simulink model "SolarPackBuckConverter"  (R2024b)
settings: Solver=VariableStepAuto  StartTime=0.0  StopTime=0.1  RelTol=1e-3
values from neighbouring files (symbols this model uses):
  C1_actual = 470e-6    (= 0.00047)    [Buck_Design.m]
  C1_esr = 50e-3    (= 0.05)    [Buck_Design.m]
  C2_actual = 470e-6    (= 0.00047)    [Buck_Design.m]
  C2_esr = 50e-3    (= 0.05)    [Buck_Design.m]
  D1 = Vstage / Vg    (= 0.190476190476)    [Buck_Design.m]
  D2 = V / Vstage    (= 0.175)    [Buck_Design.m]
  L1_actual = 270e-6    (= 0.00027)    [Buck_Design.m]
  L1_esr = 14e-3    (= 0.014)    [Buck_Design.m]
  L2_actual = 12e-6    (= 1.2e-05)    [Buck_Design.m]
  L2_esr = 2.08e-3    (= 0.00208)    [Buck_Design.m]
  Rbat = 0.008    [Buck_Design.m]
  Rlimit = 0.1    [Buck_Design.m]
  RlimitPass = 0.1    [Buck_Design.m]
  Vg = 420    [Buck_Design.m]
undefined symbols (not defined in the file or in its folder): Acid, C_actual, Lead
libraries: spsCurrentMeasurementLib x7, spsVoltageMeasurementLib x7, spsSeriesRLCBranchLib x6, spsMosfetLib x4, spsPWMGeneratorDCDCLib x4, spsDiodeLib x3, slpidlib x2, spsBatteryLib x1, spsControlledVoltageSourceLib x1, spsGroundLib x1, spsSeriesRLCLoadLib x1, sps_lib x1
settings Model: Creator=izakd  LastModifiedBy=izakd
settings SolverCC: AllowMultiTaskInputOutput=on  ZeroCrossControl=EnableAll  ZeroCrossAlgorithm=Adaptive  PositivePriorityOrder=on  AutoInsertRateTranBlk=on
settings DebuggingCC: MaskedZcDiagnostic=none  IgnoredZcDiagnostic=none

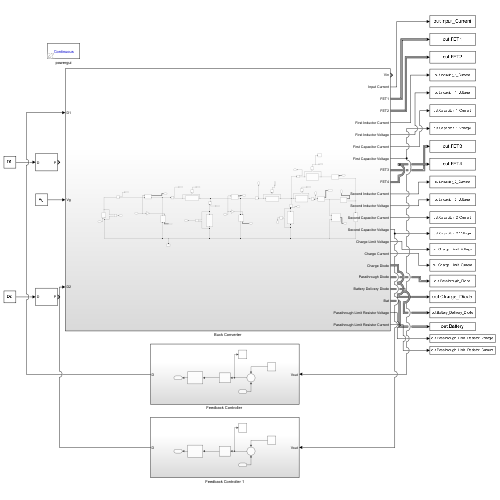
[thumbnail: Simulink's stored preview of the top-level diagram]
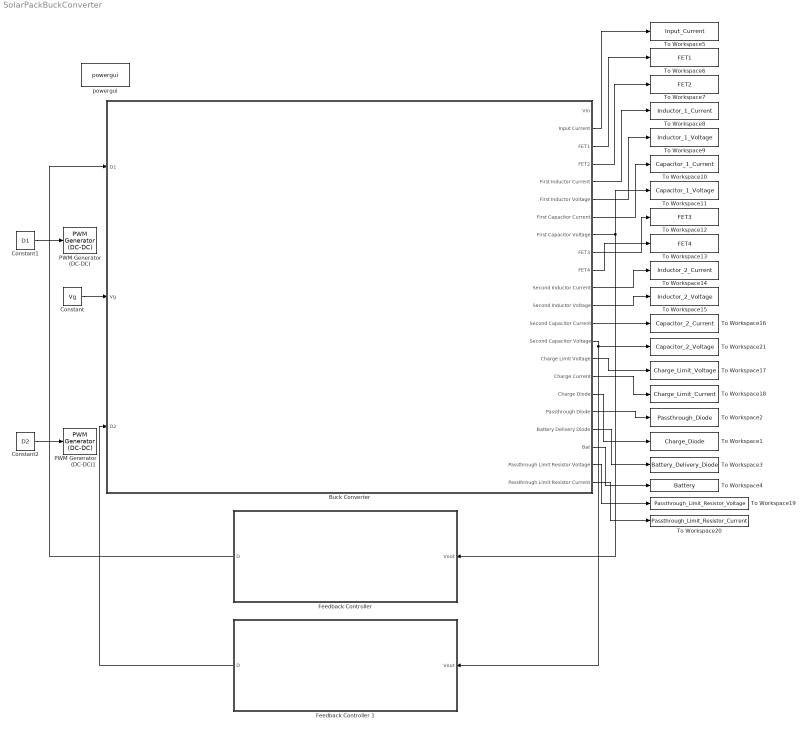
== system SolarPackBuckConverter ==
  Buck Converter : Subsystem
  Constant : Constant  Value=Vg
  Constant1 : Constant  Value=D1
  Constant2 : Constant  Value=D2
  "Feedback Controller " : Subsystem
  Feedback Controller 1 : Subsystem
  PWM Generator (DC-DC) : spsPWMGeneratorDCDCLib/PWM Generator (DC-DC)  Fsw=F  Ts=0
  PWM Generator (DC-DC)1 : spsPWMGeneratorDCDCLib/PWM Generator (DC-DC)  Fsw=F  Ts=0
  To Workspace1 : ToWorkspace  VariableName=Charge_Diode  SaveFormat=Timeseries  SampleTime=-1
  To Workspace10 : ToWorkspace  VariableName=Capacitor_1_Current  SaveFormat=Timeseries  SampleTime=-1
  To Workspace11 : ToWorkspace  VariableName=Capacitor_1_Voltage  SaveFormat=Timeseries  SampleTime=-1
  To Workspace12 : ToWorkspace  VariableName=FET3  SaveFormat=Timeseries  SampleTime=-1
  To Workspace13 : ToWorkspace  VariableName=FET4  SaveFormat=Timeseries  SampleTime=-1
  To Workspace14 : ToWorkspace  VariableName=Inductor_2_Current  SaveFormat=Timeseries  SampleTime=-1
  To Workspace15 : ToWorkspace  VariableName=Inductor_2_Voltage  SaveFormat=Timeseries  SampleTime=-1
  To Workspace16 : ToWorkspace  VariableName=Capacitor_2_Current  SaveFormat=Timeseries  SampleTime=-1
  To Workspace17 : ToWorkspace  VariableName=Charge_Limit_Voltage  SaveFormat=Timeseries  SampleTime=-1
  To Workspace18 : ToWorkspace  VariableName=Charge_Limit_Current  SaveFormat=Timeseries  SampleTime=-1
  To Workspace19 : ToWorkspace  VariableName=Passthrough_Limit_Resistor_Voltage  SaveFormat=Timeseries  SampleTime=-1
  To Workspace2 : ToWorkspace  VariableName=Passthrough_Diode  SaveFormat=Timeseries  SampleTime=-1
  To Workspace20 : ToWorkspace  VariableName=Passthrough_Limit_Resistor_Current  SaveFormat=Timeseries  SampleTime=-1
  To Workspace21 : ToWorkspace  VariableName=Capacitor_2_Voltage  SaveFormat=Timeseries  SampleTime=-1
  To Workspace3 : ToWorkspace  VariableName=Battery_Delivery_Diode  SaveFormat=Timeseries  SampleTime=-1
  To Workspace4 : ToWorkspace  VariableName=Battery  SaveFormat=Timeseries  SampleTime=-1
  To Workspace5 : ToWorkspace  VariableName=Input_Current  SaveFormat=Timeseries  SampleTime=-1
  To Workspace6 : ToWorkspace  VariableName=FET1  SaveFormat=Timeseries  SampleTime=-1
  To Workspace7 : ToWorkspace  VariableName=FET2  SaveFormat=Timeseries  SampleTime=-1
  To Workspace8 : ToWorkspace  VariableName=Inductor_1_Current  SaveFormat=Timeseries  SampleTime=-1
  To Workspace9 : ToWorkspace  VariableName=Inductor_1_Voltage  SaveFormat=Timeseries  SampleTime=-1
  powergui : sps_lib/powergui  Priority=1  SimulationMode=Continuous  SampleTime=50e-6  frequency=60  Iterations=50  frequencyindice=0  Pbase=100e6  ErrMax=1e-4  UnitsV=kV  UnitsW=MW  buscounter=0  FunctionMessages=off  echomessages=off  EnableUseOfTLC=off  CurrentSourceSwitches=off  DisableSnubberDevices=off  DisableRonSwitches=off  DisableVfSwitches=off  DisplayEquations=off  AutomaticDiscreteSolvers=off  SolverType=Tustin/Backward Euler (TBE)  Interpol=off  ExternalGateDelay=off  methode=off  Ts=100  x0status=blocks  SPID=on  SwTol=0  HookPort=off  NonlinearTolerance=1e-4  nMaxIteration=100  ContinueOnMaxIteration=off  RestoreLinks=warning  ResistiveCurrentMeasurement=off  Frange=[0:2:500]  Ylog=off  Xlog=on  ShowGrid=off  save=off  variable=ZData  structure=0  ZoomFFT=off  StartTime=0.0  cycles=1  DisplayStyle=1  fundamental=60  FreqAxis=off  MaxFrequency=1000  frequencyindicesteady=1  RmsSteady=1  display=off
  wires:
  Constant/1 -> Buck Converter/2(Vg)
  Buck Converter/2(Input Current) -> To Workspace5/1
  Buck Converter/8(First Capacitor Voltage) -> To Workspace11/1, "Feedback Controller "/1(Vout)
  Buck Converter/14(Second Capacitor Voltage) -> To Workspace21/1, Feedback Controller 1/1(Vout)
  Buck Converter/17(Charge Diode) -> To Workspace1/1
  Buck Converter/18(Passthrough Diode) -> To Workspace2/1
  Buck Converter/19(Battery Delivery Diode) -> To Workspace3/1
  Buck Converter/20(Bat) -> To Workspace4/1
  Constant1/1 -> PWM Generator (DC-DC)/1
  Constant2/1 -> PWM Generator (DC-DC)1/1
  "Feedback Controller "/1(D) -> Buck Converter/1(D1)
  Feedback Controller 1/1(D) -> Buck Converter/3(D2)
  Buck Converter/3(FET1) -> To Workspace6/1
  Buck Converter/4(FET2) -> To Workspace7/1
  Buck Converter/5(First Inductor Current) -> To Workspace8/1
  Buck Converter/6(First Inductor Voltage) -> To Workspace9/1
  Buck Converter/7(First Capacitor Current) -> To Workspace10/1
  Buck Converter/9(FET3) -> To Workspace12/1
  Buck Converter/10(FET4) -> To Workspace13/1
  Buck Converter/11(Second Inductor Current) -> To Workspace14/1
  Buck Converter/12(Second Inductor Voltage) -> To Workspace15/1
  Buck Converter/13(Second Capacitor Current) -> To Workspace16/1
  Buck Converter/15(Charge Limit Voltage) -> To Workspace17/1
  Buck Converter/21(Passthrough Limit Resistor Voltage) -> To Workspace19/1
  Buck Converter/22(Passthrough Limit Resistor Current) -> To Workspace20/1
  Buck Converter/16(Charge Current) -> To Workspace18/1

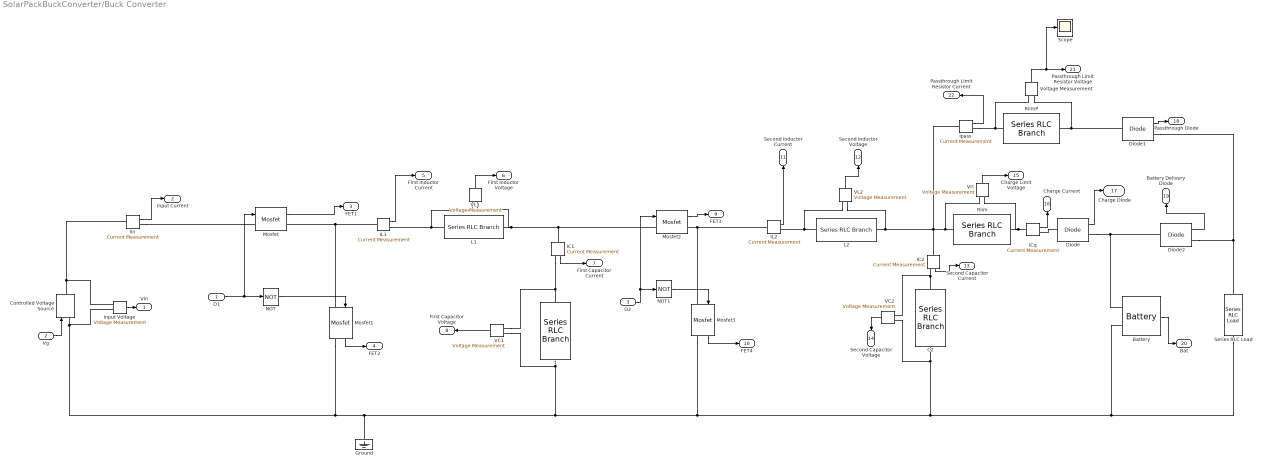
== system SolarPackBuckConverter/Buck Converter ==
  D1 : Inport
  Vg : Inport  Port=2
  D2 : Inport  Port=3
  1 : spsSeriesRLCBranchLib/Series RLC Branch  LConnTagsString=__new0  RConnTagsString=__new0  BranchType=RC  Resistance=C1_esr  Inductance=1e-3  SetiL0=off  InitialCurrent=0  Capacitance=C1_actual  Setx0=off  InitialVoltage=0  Measurements=None
  Battery : spsBatteryLib/Battery  BatType=Lead-Acid  NomV=12  NomQ=50  SOC=SOC  Batt_Tr=0.01  PresetModel=off  MaxQ=52.0833  MinV=9  FullV=13.0658  Dis_rate=10  R=Rbat  Normal_OP=15.5139  expZone="[12.2171     0.166667]"
  C2 : spsSeriesRLCBranchLib/Series RLC Branch  LConnTagsString=__new0  RConnTagsString=__new0  BranchType=RC  Resistance=C2_esr  Inductance=1e-3  SetiL0=off  InitialCurrent=0  Capacitance=C2_actual  Setx0=off  InitialVoltage=0  Measurements=None
  Controlled Voltage Source : spsControlledVoltageSourceLib/Controlled Voltage Source  Initialize=on  Source_Type=DC  Amplitude=0  Phase=0  Frequency=0  Measurements=Voltage
  Diode : spsDiodeLib/Diode  Ron=Rdiode_Charge  Lon=0  Vf=Vfdiode_Charge  IC=0  UseSnubber=0  Rs=500  Cs=250e-9  Measurements=on
  Diode1 : spsDiodeLib/Diode  Ron=Rdiode  Lon=0  Vf=Vfdiode  IC=0  UseSnubber=0  Rs=500  Cs=250e-9  Measurements=on
  Diode2 : spsDiodeLib/Diode  Ron=Rdiode  Lon=0  Vf=Vfdiode  IC=0  UseSnubber=0  Rs=500  Cs=250e-9  Measurements=on
  Ground : spsGroundLib/Ground  LConnTagsString=a
  IC1 : spsCurrentMeasurementLib/Current Measurement  PhasorSimulation=off  OutputType=Complex  PSBequivalent=0
  IC2 : spsCurrentMeasurementLib/Current Measurement  PhasorSimulation=off  OutputType=Complex  PSBequivalent=0
  ICq : spsCurrentMeasurementLib/Current Measurement  PhasorSimulation=off  OutputType=Complex  PSBequivalent=0
  IL1 : spsCurrentMeasurementLib/Current Measurement  PhasorSimulation=off  OutputType=Complex  PSBequivalent=0
  IL2 : spsCurrentMeasurementLib/Current Measurement  PhasorSimulation=off  OutputType=Complex  PSBequivalent=0
  Iin : spsCurrentMeasurementLib/Current Measurement  PhasorSimulation=off  OutputType=Complex  PSBequivalent=0
  Input Voltage : spsVoltageMeasurementLib/Voltage Measurement  PhasorSimulation=off  OutputType=Complex  PSBequivalent=0
  Ipass : spsCurrentMeasurementLib/Current Measurement  PhasorSimulation=off  OutputType=Complex  PSBequivalent=0
  L1 : spsSeriesRLCBranchLib/Series RLC Branch  LConnTagsString=__new0  RConnTagsString=__new0  BranchType=RL  Resistance=L1_esr  Inductance=L1_actual  SetiL0=off  InitialCurrent=0  Capacitance=1e-6  Setx0=off  InitialVoltage=0  Measurements=None
  L2 : spsSeriesRLCBranchLib/Series RLC Branch  LConnTagsString=__new0  RConnTagsString=__new0  BranchType=RL  Resistance=L2_esr  Inductance=L2_actual  SetiL0=off  InitialCurrent=0  Capacitance=1e-6  Setx0=off  InitialVoltage=0  Measurements=None
  Mosfet{,1..3} (4 alike) : spsMosfetLib/Mosfet  Ron=Ron  Lon=0  Rd=0.01  Vfd=Vf  IC=0  Rs=1e5  Cs=inf  Measurements=on
  NOT : Logic  Operator=NOT  IconShape=distinctive  AllPortsSameDT=off  OutDataTypeStr=boolean
  NOT1 : Logic  Operator=NOT  IconShape=distinctive  AllPortsSameDT=off  OutDataTypeStr=boolean
  Rlim : spsSeriesRLCBranchLib/Series RLC Branch  LConnTagsString=__new0  RConnTagsString=__new0  BranchType=R  Resistance=Rlimit  Inductance=1e-3  SetiL0=off  InitialCurrent=0  Capacitance=C_actual  Setx0=off  InitialVoltage=0  Measurements=None
  RlimP : spsSeriesRLCBranchLib/Series RLC Branch  LConnTagsString=__new0  RConnTagsString=__new0  BranchType=R  Resistance=RlimitPass  Inductance=1e-3  SetiL0=off  InitialCurrent=0  Capacitance=C_actual  Setx0=off  InitialVoltage=0  Measurements=None
  Scope : Scope
  Series RLC Load : spsSeriesRLCLoadLib/Series RLC Load  LConnTagsString=a  RConnTagsString=__new0  NominalVoltage=13.2  NominalFrequency=8e7  ActivePower=Pload  InductivePower=0  CapacitivePower=0  Setx0=off  InitialVoltage=0  SetiL0=off  InitialCurrent=0  Measurements=None  LoadType=constant Z
  VC1 : spsVoltageMeasurementLib/Voltage Measurement  PhasorSimulation=off  OutputType=Complex  PSBequivalent=0
  VC2 : spsVoltageMeasurementLib/Voltage Measurement  PhasorSimulation=off  OutputType=Complex  PSBequivalent=0
  VL1 : spsVoltageMeasurementLib/Voltage Measurement  PhasorSimulation=off  OutputType=Complex  PSBequivalent=0
  VL2 : spsVoltageMeasurementLib/Voltage Measurement  PhasorSimulation=off  OutputType=Complex  PSBequivalent=0
  Voltage Measurement : spsVoltageMeasurementLib/Voltage Measurement  PhasorSimulation=off  OutputType=Complex  PSBequivalent=0
  Vrl : spsVoltageMeasurementLib/Voltage Measurement  PhasorSimulation=off  OutputType=Complex  PSBequivalent=0
  Vin : Outport
  Input Current : Outport  Port=2
  FET1 : Outport  Port=3
  FET2 : Outport  Port=4
  First Inductor Current : Outport  Port=5
  First Inductor Voltage : Outport  Port=6
  First Capacitor Current : Outport  Port=7
  First Capacitor Voltage : Outport  Port=8
  FET3 : Outport  Port=9
  FET4 : Outport  Port=10
  Second Inductor Current : Outport  Port=11
  Second Inductor Voltage : Outport  Port=12
  Second Capacitor Current : Outport  Port=13
  Second Capacitor Voltage : Outport  Port=14
  Charge Limit Voltage : Outport  Port=15
  Charge Current : Outport  Port=16
  Charge Diode : Outport  Port=17
  Passthrough Diode : Outport  Port=18
  Battery Delivery Diode : Outport  Port=19
  Bat : Outport  Port=20
  Passthrough Limit Resistor Voltage : Outport  Port=21
  Passthrough Limit Resistor Current : Outport  Port=22
  wires:
  D1/1 -> NOT/1, Mosfet/1
  Mosfet1/1 -> FET2/1
  Mosfet/1 -> FET1/1
  Vg/1 -> Controlled Voltage Source/1
  IC1/1 -> First Capacitor Current/1
  NOT/1 -> Mosfet1/1
  VL1/1 -> First Inductor Voltage/1
  IL1/1 -> First Inductor Current/1
  VC1/1 -> First Capacitor Voltage/1
  Input Voltage/1 -> Vin/1
  Iin/1 -> Input Current/1
  Mosfet2/1 -> FET3/1
  Mosfet3/1 -> FET4/1
  D2/1 -> Mosfet2/1, NOT1/1
  NOT1/1 -> Mosfet3/1
  IL2/1 -> Second Inductor Current/1
  VL2/1 -> Second Inductor Voltage/1
  IC2/1 -> Second Capacitor Current/1
  VC2/1 -> Second Capacitor Voltage/1
  Vrl/1 -> Charge Limit Voltage/1
  ICq/1 -> Charge Current/1
  Diode/1 -> Charge Diode/1
  Diode1/1 -> Passthrough Diode/1
  Diode2/1 -> Battery Delivery Diode/1
  Battery/1 -> Bat/1
  Voltage Measurement/1 -> Scope/1, Passthrough Limit Resistor Voltage/1
  Ipass/1 -> Passthrough Limit Resistor Current/1
  connections:
  Iin/RConn1 -- Mosfet/LConn1
  VL1/LConn1 -- IL1/RConn1 -- L1/LConn1
  Controlled Voltage Source/RConn1 -- Iin/LConn1 -- Input Voltage/LConn1
  IL1/LConn1 -- Mosfet1/LConn1 -- Mosfet/RConn1
  VC1/LConn1 -- IC1/RConn1 -- 1/LConn1
  L1/RConn1 -- VL1/LConn2 -- Mosfet2/LConn1 -- IC1/LConn1
  Mosfet3/LConn1 -- IL2/LConn1 -- Mosfet2/RConn1
  L2/LConn1 -- IL2/RConn1 -- VL2/LConn1
  C2/LConn1 -- VC2/LConn1 -- IC2/RConn1
  IC2/LConn1 -- Ipass/LConn1 -- Vrl/LConn1 -- Rlim/RConn1 -- VL2/LConn2 -- L2/RConn1
  Series RLC Load/LConn1 -- Diode1/RConn1 -- Diode2/RConn1
  Diode/RConn1 -- Diode2/LConn1 -- Battery/LConn1
  ICq/LConn1 -- Vrl/LConn2 -- Rlim/LConn1
  Diode/LConn1 -- ICq/RConn1
  Mosfet1/RConn1 -- Series RLC Load/RConn1 -- Battery/LConn2 -- C2/RConn1 -- VC2/LConn2 -- Mosfet3/RConn1 -- 1/RConn1 -- VC1/LConn2 -- Ground/LConn1 -- Input Voltage/LConn2 -- Controlled Voltage Source/LConn1
  Diode1/LConn1 -- Voltage Measurement/LConn2 -- RlimP/LConn1
  RlimP/RConn1 -- Voltage Measurement/LConn1 -- Ipass/RConn1

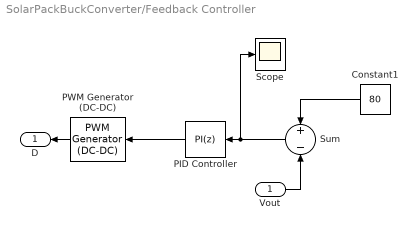
== system SolarPackBuckConverter/Feedback Controller  ==
  Vout : Inport
  Constant1 : Constant  Value=80
  PID Controller : slpidlib/PID Controller  Controller=PI  Form=Parallel  TimeDomain=Discrete-time  UseExternalTs=off  SampleTime=1/400e3  IntegratorMethod=Forward Euler  FilterMethod=Forward Euler  ControllerParametersSource=internal  P=0.01  I=5  UseKiTs=off  D=0  UseExternalDerivativeSource=off  N=100  UseFilter=on  TunerSelectOption=Transfer Function Based (PID Tuner App)  InitialConditionSource=internal  InitialConditionForIntegrator=0  InitialConditionForFilter=0  DifferentiatorICPrevScaledInput=0  ExternalReset=none  TrackingMode=off  Kt=1  LimitOutput=off  SatLimitsSource=internal  UpperSaturationLimit=inf  LowerSaturationLimit=-inf  LinearizeAsGain=on  AntiWindupMode=none  Kb=1  LimitIntegrator=off  UpperIntegratorSaturationLimit=inf  LowerIntegratorSaturationLimit=-inf  POutMin=[]  POutMax=[]  IOutMin=[]  IOutMax=[]  DOutMin=[]  DOutMax=[]  NOutMin=[]  NOutMax=[]  SumOutMin=[]  SumOutMax=[]  SaturationOutMin=[]  SaturationOutMax=[]  PParamMin=[]  PParamMax=[]  IParamMin=[]  IParamMax=[]  DParamMin=[]  DParamMax=[]  NParamMin=[]  NParamMax=[]  KbParamMin=[]  KbParamMax=[]  KtParamMin=[]  KtParamMax=[]  KbOutMin=[]  KbOutMax=[]  KtOutMin=[]  KtOutMax=[]  IntegratorOutMin=[]  IntegratorOutMax=[]  FilterOutMin=[]  FilterOutMax=[]  SumI1OutMin=[]  SumI1OutMax=[]  SumI2OutMin=[]  SumI2OutMax=[]  SumI3OutMin=[]  SumI3OutMax=[]  SumI4OutMin=[]  SumI4OutMax=[]  SumDOutMin=[]  SumDOutMax=[]  DifferentiatorOutMin=[]  DifferentiatorOutMax=[]  FilterDiffOutCoefMin=[]  FilterDiffOutCoefMax=[]  ReciprocalOutMin=[]  ReciprocalOutMax=[]  SumDenOutMin=[]  SumDenOutMax=[]  SumNumOutMin=[]  SumNumOutMax=[]  DivideOutMin=[]  DivideOutMax=[]  UdiffTsProdOutMin=[]  UdiffTsProdOutMax=[]  NTsProdOutMin=[]  NTsProdOutMax=[]  UintegralTsProdOutMin=[]  UintegralTsProdOutMax=[]  UngainTsProdOutMin=[]  UngainTsProdOutMax=[]  ClampingZeroOutDataTypeStr=Inherit: Inherit via back propagation  ClampingZeroOutMin=[]  ClampingZeroOutMax=[]  FilterDenConstantOutDataTypeStr=Inherit: Inherit via back propagation  FilterDenConstantOutMin=[]  FilterDenConstantOutMax=[]  PCopyOutDataTypeStr=Inherit: Inherit via back propagation  PCopyOutMin=[]  PCopyOutMax=[]  NCopyOutDataTypeStr=Inherit: Inherit via back propagation  NCopyOutMin=[]  NCopyOutMax=[]  IntegratorContinuousStateAttributes=''  IntegratorStateMustResolveToSignalObject=off  IntegratorRTWStateStorageClass=Auto  FilterContinuousStateAttributes=''  FilterStateMustResolveToSignalObject=off  FilterRTWStateStorageClass=Auto  ParallelPVariant=InternalParameters  IdealPVariant=Disabled  IVariant=InternalParameters  DVariant=Disabled  IntegratorVariant=Discrete  SatVariant=Disabled  AWVariant=Passthrough  PCopyVariant=Disabled  TRVariant=Disabled  FdbkBlocksVariant=Forward  IdealPFdbkVariant=Disabled  SatFdbkVariant=Disabled  DerivativeFilterVariant=Disabled  NVariant=Disabled  NCopyVariant=Disabled_SignalSpec  FilterICVariant=Disabled  IntegratorICVariant=InternalICs  ExternalResetVariant=Disabled  TRSumVariant=Passthrough  SumFdbkVariant=Disabled  SumVariant=Sum_PI  TsampFilterVariant=InternalTs  TsampNgainVariant=Passthrough  TsampIntegralVariant=Disabled_SignalSpec  ExternalSaturationOutDataTypeStr=Inherit: Same as second input  DerivativeSourceVariant=Disabled  PreIntVariant=InternalPreInt
  PWM Generator (DC-DC) : spsPWMGeneratorDCDCLib/PWM Generator (DC-DC)  Fsw=F  Ts=0
  Scope : Scope
  Sum : Sum  Inputs=+-
  D : Outport
  wires:
  PID Controller/1 -> PWM Generator (DC-DC)/1
  Vout/1 -> Sum/2
  Constant1/1 -> Sum/1
  Sum/1 -> Scope/1, PID Controller/1
  PWM Generator (DC-DC)/1 -> D/1

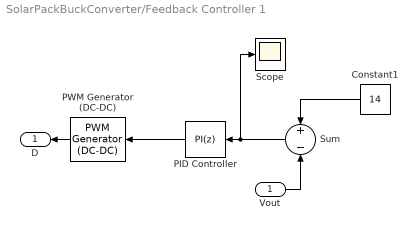
== system SolarPackBuckConverter/Feedback Controller 1 ==
  Vout : Inport
  Constant1 : Constant  Value=14
  PID Controller : slpidlib/PID Controller  Controller=PI  Form=Parallel  TimeDomain=Discrete-time  UseExternalTs=off  SampleTime=1/400e3  IntegratorMethod=Forward Euler  FilterMethod=Forward Euler  ControllerParametersSource=internal  P=0.01  I=5  UseKiTs=off  D=0  UseExternalDerivativeSource=off  N=100  UseFilter=on  TunerSelectOption=Transfer Function Based (PID Tuner App)  InitialConditionSource=internal  InitialConditionForIntegrator=0  InitialConditionForFilter=0  DifferentiatorICPrevScaledInput=0  ExternalReset=none  TrackingMode=off  Kt=1  LimitOutput=off  SatLimitsSource=internal  UpperSaturationLimit=inf  LowerSaturationLimit=-inf  LinearizeAsGain=on  AntiWindupMode=none  Kb=1  LimitIntegrator=off  UpperIntegratorSaturationLimit=inf  LowerIntegratorSaturationLimit=-inf  POutMin=[]  POutMax=[]  IOutMin=[]  IOutMax=[]  DOutMin=[]  DOutMax=[]  NOutMin=[]  NOutMax=[]  SumOutMin=[]  SumOutMax=[]  SaturationOutMin=[]  SaturationOutMax=[]  PParamMin=[]  PParamMax=[]  IParamMin=[]  IParamMax=[]  DParamMin=[]  DParamMax=[]  NParamMin=[]  NParamMax=[]  KbParamMin=[]  KbParamMax=[]  KtParamMin=[]  KtParamMax=[]  KbOutMin=[]  KbOutMax=[]  KtOutMin=[]  KtOutMax=[]  IntegratorOutMin=[]  IntegratorOutMax=[]  FilterOutMin=[]  FilterOutMax=[]  SumI1OutMin=[]  SumI1OutMax=[]  SumI2OutMin=[]  SumI2OutMax=[]  SumI3OutMin=[]  SumI3OutMax=[]  SumI4OutMin=[]  SumI4OutMax=[]  SumDOutMin=[]  SumDOutMax=[]  DifferentiatorOutMin=[]  DifferentiatorOutMax=[]  FilterDiffOutCoefMin=[]  FilterDiffOutCoefMax=[]  ReciprocalOutMin=[]  ReciprocalOutMax=[]  SumDenOutMin=[]  SumDenOutMax=[]  SumNumOutMin=[]  SumNumOutMax=[]  DivideOutMin=[]  DivideOutMax=[]  UdiffTsProdOutMin=[]  UdiffTsProdOutMax=[]  NTsProdOutMin=[]  NTsProdOutMax=[]  UintegralTsProdOutMin=[]  UintegralTsProdOutMax=[]  UngainTsProdOutMin=[]  UngainTsProdOutMax=[]  ClampingZeroOutDataTypeStr=Inherit: Inherit via back propagation  ClampingZeroOutMin=[]  ClampingZeroOutMax=[]  FilterDenConstantOutDataTypeStr=Inherit: Inherit via back propagation  FilterDenConstantOutMin=[]  FilterDenConstantOutMax=[]  PCopyOutDataTypeStr=Inherit: Inherit via back propagation  PCopyOutMin=[]  PCopyOutMax=[]  NCopyOutDataTypeStr=Inherit: Inherit via back propagation  NCopyOutMin=[]  NCopyOutMax=[]  IntegratorContinuousStateAttributes=''  IntegratorStateMustResolveToSignalObject=off  IntegratorRTWStateStorageClass=Auto  FilterContinuousStateAttributes=''  FilterStateMustResolveToSignalObject=off  FilterRTWStateStorageClass=Auto  ParallelPVariant=InternalParameters  IdealPVariant=Disabled  IVariant=InternalParameters  DVariant=Disabled  IntegratorVariant=Discrete  SatVariant=Disabled  AWVariant=Passthrough  PCopyVariant=Disabled  TRVariant=Disabled  FdbkBlocksVariant=Forward  IdealPFdbkVariant=Disabled  SatFdbkVariant=Disabled  DerivativeFilterVariant=Disabled  NVariant=Disabled  NCopyVariant=Disabled_SignalSpec  FilterICVariant=Disabled  IntegratorICVariant=InternalICs  ExternalResetVariant=Disabled  TRSumVariant=Passthrough  SumFdbkVariant=Disabled  SumVariant=Sum_PI  TsampFilterVariant=InternalTs  TsampNgainVariant=Passthrough  TsampIntegralVariant=Disabled_SignalSpec  ExternalSaturationOutDataTypeStr=Inherit: Same as second input  DerivativeSourceVariant=Disabled  PreIntVariant=InternalPreInt
  PWM Generator (DC-DC) : spsPWMGeneratorDCDCLib/PWM Generator (DC-DC)  Fsw=F  Ts=0
  Scope : Scope
  Sum : Sum  Inputs=+-
  D : Outport
  wires:
  PID Controller/1 -> PWM Generator (DC-DC)/1
  Vout/1 -> Sum/2
  Constant1/1 -> Sum/1
  Sum/1 -> Scope/1, PID Controller/1
  PWM Generator (DC-DC)/1 -> D/1
